simulink model "simulation_strecke"  (Simulink 7.0)
settings: Solver=ode45  StartTime=0.0  StopTime=10.0  RelTol=1e-3
settings Model: Creator=Matze  LastModifiedBy=Matze

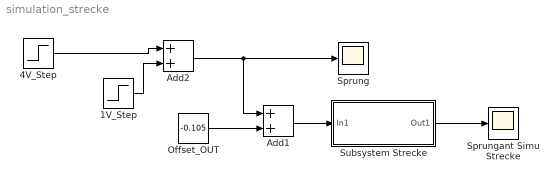
== system simulation_strecke ==
  1V_Step : Step  Time=3.0  SampleTime=0
  4V_Step : Step  After=4  SampleTime=0
  Add1 : Sum  OutDataType=sfix(16)  OutScaling=2^-10
  Add2 : Sum  OutDataType=sfix(16)  OutScaling=2^-10
  Offset_OUT : Constant  Value=-0.105  OutDataType=sfix(16)  OutScaling=2^0
  Sprung : Scope
      settings: TimeRange=10  YMin=0
  Sprungant Simu Strecke : Scope
  Subsystem Strecke : Subsystem
  wires:
  Subsystem Strecke/1(Out1) -> Sprungant Simu Strecke/1
  4V_Step/1 -> Add2/1
  Offset_OUT/1 -> Add1/2
  Add2/1 -> Add1/1, Sprung/1
  1V_Step/1 -> Add2/2
  Add1/1 -> Subsystem Strecke/1(In1)

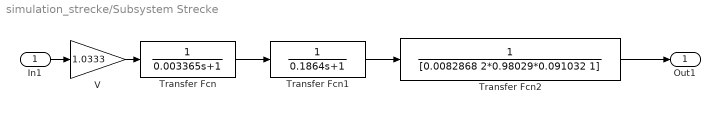
== system simulation_strecke/Subsystem Strecke ==
  In1 : Inport  OutDataType=sfix(16)  OutScaling=2^0
  Transfer Fcn : TransferFcn  Denominator=[0.003365 1]
  Transfer Fcn1 : TransferFcn  Denominator=[0.1864 1]
  Transfer Fcn2 : TransferFcn  Denominator=[0.0082868 2*0.98029*0.091032 1]
  V : Gain  Gain=1.0333  ParameterDataType=sfix(16)  ParameterScaling=2^0  OutDataType=sfix(16)  OutScaling=2^0
  Out1 : Outport  OutDataType=sfix(16)  OutScaling=2^0
  wires:
  In1/1 -> V/1
  V/1 -> Transfer Fcn/1
  Transfer Fcn/1 -> Transfer Fcn1/1
  Transfer Fcn1/1 -> Transfer Fcn2/1
  Transfer Fcn2/1 -> Out1/1
